simulink model "cte_mec"  (Simulink 6.1)
settings: Solver=ode23tb  SolverMode=SingleTasking  StartTime=0.0  StopTime=20  MaxStep=1e-4
libraries: powerlib2 x2
settings Model: LastModifiedBy=Administrador  ExtModeTrigMode=oneshot  ExtModeArmWhenConnect=off
settings DataIOCC: LimitDataPoints=off  SaveFinalState=on  SaveOutput=off  SaveTime=off  SignalLoggingName=sigsOut
settings OptimizationCC: BlockReduction=off  BooleanDataType=off  InlineInvariantSignals=off
settings DebuggingCC: UnconnectedInputMsg=none  UnconnectedOutputMsg=none
settings HardwareCC: TargetUnknown=on
settings RTWCC: TemplateMakefile=grt_unix.tmf

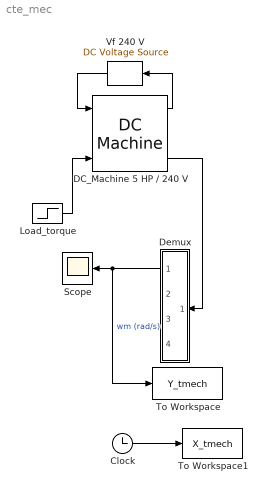
== system cte_mec ==
  Clock : Clock
      settings: Decimation=10
  DC_Machine 5 HP / 240 V : powerlib2/Machines/DC Machine  RLa=[0.5 0.01]  RLf="[240  0]"  Laf=1.23  J=0.05  Bm=0.02  Tf=0  w0=1e-1  PSBOutputType=110
  Demux : Subsystem  Orientation=left
  "Load_torque " : Step  Time=1e-5  After=-5  SampleTime=0
  Scope : Scope
      settings: YMin=0  YMax=255
  To Workspace : ToWorkspace  VariableName=Y_tmech  SampleTime=-1  SaveFormat=Array
  To Workspace1 : ToWorkspace  VariableName=X_tmech  SampleTime=-1  SaveFormat=Array
  Vf 240 V : powerlib2/Electrical Sources/DC Voltage Source  Tag=PoWeRsYsTeMbLoCk  Orientation=left  V=240  mesure=None  PSBOutputType=1
  wires:
  Vf 240 V/1 -> DC_Machine 5 HP / 240 V/1
  DC_Machine 5 HP / 240 V/1 -> Vf 240 V/1
  DC_Machine 5 HP / 240 V/3 -> Demux/1(m)
  "Load_torque "/1 -> DC_Machine 5 HP / 240 V/3
  Demux/1(wm) -> Scope/1, To Workspace/1  "wm (rad/s)"
  Clock/1 -> To Workspace1/1

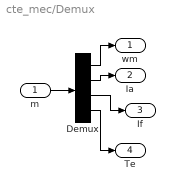
== system cte_mec/Demux ==
  m : Inport  Port=1  LatchInput=off
  Demux : Demux
  wm : Outport
  Ia : Outport  Port=2
  If : Outport  Port=3
  Te : Outport  Port=4
  wires:
  Demux/1 -> wm/1
  Demux/2 -> Ia/1
  m/1 -> Demux/1
  Demux/3 -> If/1
  Demux/4 -> Te/1
